simulink model "orbit"  (R2025b)
settings: Solver=ode45  StartTime=0.0  StopTime=endTime  FixedStep=1/60  MaxStep=10  RelTol=1e-10  AbsTol=1e-10
undefined symbols (not defined in the file or in its folder): panelY
libraries: aerolibutil x9, aerolibsatdyn x3, simulink_extras x2
settings Model: Creator=The MathWorks, Inc.  LastModifiedBy=axmal
settings OptimizationCC: ReuseModelBlockBuffer=off
settings ModelReferenceCC: EnableRefExpFcnMdlSchedulingChecks=on
settings RTWCC: GPUComputeCapability=3.5

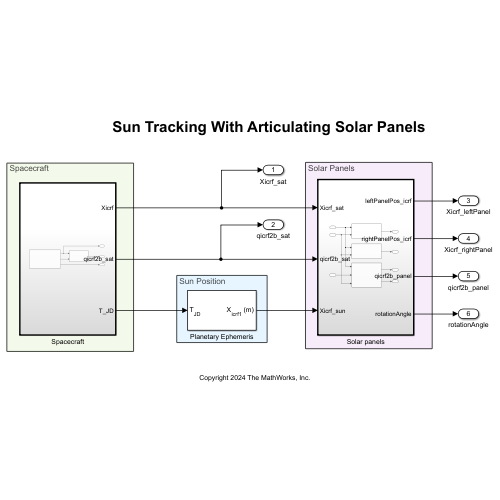
[thumbnail: Simulink's stored preview of the top-level diagram]
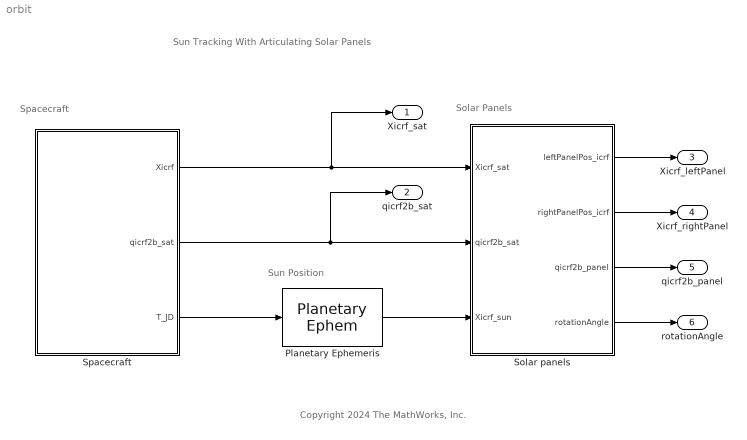
== system orbit ==
  note: Sun Position
  note: Spacecraft
  note: Sun Tracking With Articulating Solar Panels
  note: Copyright 2024 The MathWorks, Inc.
  note: Solar Panels
  Planetary Ephemeris : PlanetaryEphem  units=m,m/s  target=Sun  outputVelocity=off
  Solar panels : Subsystem  TreatAsAtomicUnit=on
  Spacecraft : Subsystem  TreatAsAtomicUnit=on
  Xicrf_sat : Outport
  qicrf2b_sat : Outport  Port=2
  Xicrf_leftPanel : Outport  Port=3
  Xicrf_rightPanel : Outport  Port=4
  qicrf2b_panel : Outport  Port=5
  rotationAngle : Outport  Port=6
  wires:
  Spacecraft/3(T_JD) -> Planetary Ephemeris/1
  Spacecraft/2(qicrf2b_sat) -> qicrf2b_sat/1, Solar panels/2(qicrf2b_sat)
  Solar panels/2(rightPanelPos_icrf) -> Xicrf_rightPanel/1
  Solar panels/3(qicrf2b_panel) -> qicrf2b_panel/1
  Spacecraft/1(Xicrf) -> Xicrf_sat/1, Solar panels/1(Xicrf_sat)
  Planetary Ephemeris/1 -> Solar panels/3(Xicrf_sun)
  Solar panels/1(leftPanelPos_icrf) -> Xicrf_leftPanel/1
  Solar panels/4(rotationAngle) -> rotationAngle/1

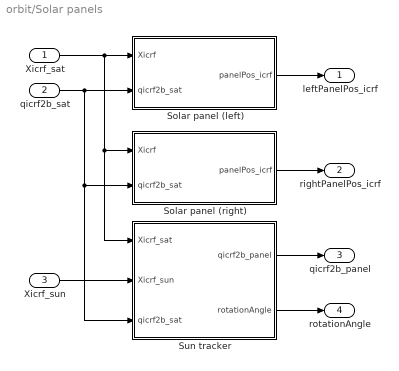
== system orbit/Solar panels ==
  Xicrf_sat : Inport
  qicrf2b_sat : Inport  Port=2
  Xicrf_sun : Inport  Port=3
  Solar panel (left) : Subsystem
  Solar panel (right) : Subsystem
  Sun tracker : Subsystem
  leftPanelPos_icrf : Outport
  rightPanelPos_icrf : Outport  Port=2
  qicrf2b_panel : Outport  Port=3
  rotationAngle : Outport  Port=4
  wires:
  Sun tracker/1(qicrf2b_panel) -> qicrf2b_panel/1
  Solar panel (right)/1(panelPos_icrf) -> rightPanelPos_icrf/1
  qicrf2b_sat/1 -> Sun tracker/3(qicrf2b_sat), Solar panel (right)/2(qicrf2b_sat), Solar panel (left)/2(qicrf2b_sat)
  Xicrf_sat/1 -> Sun tracker/1(Xicrf_sat), Solar panel (right)/1(Xicrf), Solar panel (left)/1(Xicrf)
  Solar panel (left)/1(panelPos_icrf) -> leftPanelPos_icrf/1
  Sun tracker/2(rotationAngle) -> rotationAngle/1
  Xicrf_sun/1 -> Sun tracker/2(Xicrf_sun)

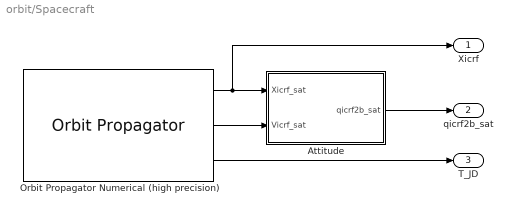
== system orbit/Spacecraft ==
  "Attitude " : Subsystem  TreatAsAtomicUnit=on
  Orbit Propagator Numerical (high precision) : OrbitPropagator  propagator=Numerical (high precision)  startDate=initialTimeJD  semiMajorAxis=semiMajorAxis  eccentricity=eccentricity  inclination=inclination  raan=rightAscensionOfAscendingNode  argPeriapsis=argumentOfPeriapsis  trueAnomaly=trueAnomaly  inertialPosition=[3649700.0 3308200.0 -4676600.0]  inertialVelocity=[-2750.8 6666.4 2573.4]  fixedPosition=[-4142689.0 -2676864.7 -4669861.6]  fixedVelocity=[1452.7 -6720.7 2568.1]  gravityModel=Point-mass  customR=3396200  customMu=4.305e13  customJ2=1.0826269e-03  customOmega=4.06125949e-3  useEOPs=off
  Xicrf : Outport
  qicrf2b_sat : Outport  Port=2
  T_JD : Outport  Port=3
  wires:
  Orbit Propagator Numerical (high precision)/3 -> T_JD/1
  Orbit Propagator Numerical (high precision)/1 -> Xicrf/1, "Attitude "/1(Xicrf_sat)
  Orbit Propagator Numerical (high precision)/2 -> "Attitude "/2(Vicrf_sat)
  "Attitude "/1(qicrf2b_sat) -> qicrf2b_sat/1

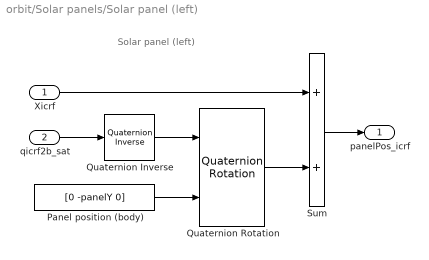
== system orbit/Solar panels/Solar panel (left) ==
  note: Solar panel (left)
  Xicrf : Inport
  qicrf2b_sat : Inport  Port=2
  Panel position (body) : Constant  Value=[0 -panelY 0]
  Quaternion Inverse : aerolibutil/Quaternion Inverse
  Quaternion Rotation : aerolibutil/Quaternion Rotation
  Sum : Sum
  panelPos_icrf : Outport
  wires:
  Quaternion Inverse/1 -> Quaternion Rotation/1
  Quaternion Rotation/1 -> Sum/2
  qicrf2b_sat/1 -> Quaternion Inverse/1
  Panel position (body)/1 -> Quaternion Rotation/2
  Xicrf/1 -> Sum/1
  Sum/1 -> panelPos_icrf/1

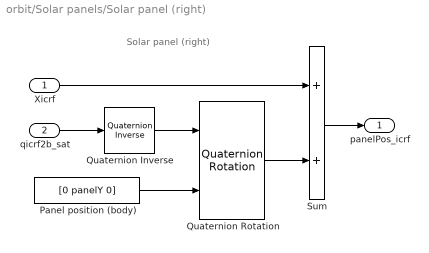
== system orbit/Solar panels/Solar panel (right) ==
  note: Solar panel (right)
  Xicrf : Inport
  qicrf2b_sat : Inport  Port=2
  Panel position (body) : Constant  Value=[0 panelY 0]
  Quaternion Inverse : aerolibutil/Quaternion Inverse
  Quaternion Rotation : aerolibutil/Quaternion Rotation
  Sum : Sum
  panelPos_icrf : Outport
  wires:
  Quaternion Inverse/1 -> Quaternion Rotation/1
  Quaternion Rotation/1 -> Sum/2
  qicrf2b_sat/1 -> Quaternion Inverse/1
  Panel position (body)/1 -> Quaternion Rotation/2
  Xicrf/1 -> Sum/1
  Sum/1 -> panelPos_icrf/1

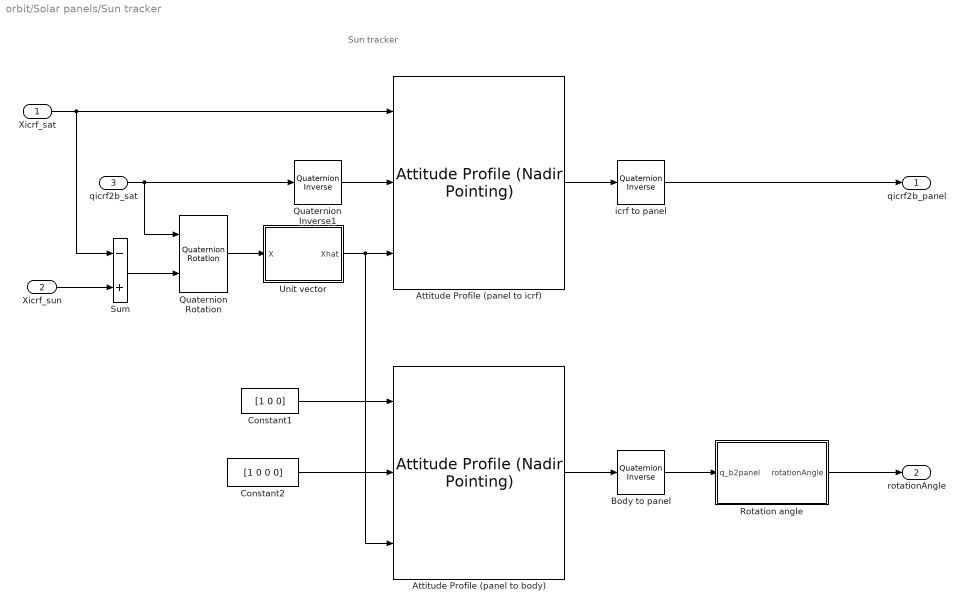
== system orbit/Solar panels/Sun tracker ==
  note: Sun tracker
  Xicrf_sat : Inport
  Xicrf_sun : Inport  Port=2
  qicrf2b_sat : Inport  Port=3
  Attitude Profile (panel to body) : aerolibsatdyn/Attitude Profile (Nadir Pointing)  outputError=off  outputFinalAttitude=on  portFrame=ICRF  pointingMode=Custom  celestialTarget=Sun  tunablePointing=off  primaryAlignmentSrc=Dialog  primaryAlignment=[0 1 0]  secondaryAlignmentSrc=Dialog  secondaryAlignment=[0 0 1]  constraintFrame=Body-frame  primaryConstraintSrc=Dialog  primaryConstraint=[0 1 0]  secondaryConstraintSrc=Port  secondaryConstraint=[0 1 0]
  Attitude Profile (panel to icrf) : aerolibsatdyn/Attitude Profile (Nadir Pointing)  outputError=off  outputFinalAttitude=on  portFrame=ICRF  pointingMode=Custom  celestialTarget=Sun  tunablePointing=off  primaryAlignmentSrc=Dialog  primaryAlignment=[0 1 0]  secondaryAlignmentSrc=Dialog  secondaryAlignment=[0 0 1]  constraintFrame=Body-frame  primaryConstraintSrc=Dialog  primaryConstraint=[0 1 0]  secondaryConstraintSrc=Port  secondaryConstraint=[0 1 0]
  Body to panel : aerolibutil/Quaternion Inverse
  Constant1 : Constant  Value=[1 0 0]
  Constant2 : Constant  Value=[1 0 0 0]
  Quaternion Inverse1 : aerolibutil/Quaternion Inverse
  Quaternion Rotation : aerolibutil/Quaternion Rotation
  Rotation angle : Subsystem
  Sum : Sum  Inputs=-+
  Unit vector : Subsystem
  icrf to panel : aerolibutil/Quaternion Inverse
  qicrf2b_panel : Outport
  rotationAngle : Outport  Port=2
  wires:
  icrf to panel/1 -> qicrf2b_panel/1
  qicrf2b_sat/1 -> Quaternion Rotation/1, Quaternion Inverse1/1
  Quaternion Inverse1/1 -> Attitude Profile (panel to icrf)/2
  Xicrf_sat/1 -> Sum/1, Attitude Profile (panel to icrf)/1
  Attitude Profile (panel to icrf)/1 -> icrf to panel/1
  Quaternion Rotation/1 -> Unit vector/1(X)
  Attitude Profile (panel to body)/1 -> Body to panel/1
  Constant1/1 -> Attitude Profile (panel to body)/1
  Unit vector/1(Xhat) -> Attitude Profile (panel to body)/3, Attitude Profile (panel to icrf)/3
  Constant2/1 -> Attitude Profile (panel to body)/2
  Body to panel/1 -> Rotation angle/1(q_b2panel)
  Rotation angle/1(rotationAngle) -> rotationAngle/1
  Xicrf_sun/1 -> Sum/2
  Sum/1 -> Quaternion Rotation/2

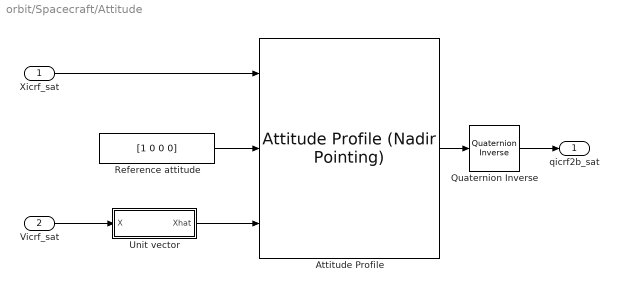
== system orbit/Spacecraft/Attitude  ==
  Xicrf_sat : Inport
  Vicrf_sat : Inport  Port=2
  Attitude Profile : aerolibsatdyn/Attitude Profile (Nadir Pointing)  outputError=off  outputFinalAttitude=on  portFrame=ICRF  pointingMode=Point at nadir  celestialTarget=Sun  tunablePointing=off  primaryAlignmentSrc=Dialog  primaryAlignment=[0 0 1]  secondaryAlignmentSrc=Dialog  secondaryAlignment=[1 0 0]  constraintFrame=ICRF  primaryConstraintSrc=Port  primaryConstraint=[1 0 0]  secondaryConstraintSrc=Port  secondaryConstraint=[0 0 1]
  Quaternion Inverse : aerolibutil/Quaternion Inverse
  Reference attitude : Constant  Value=[1 0 0 0]
  Unit vector : Subsystem
  qicrf2b_sat : Outport
  wires:
  Quaternion Inverse/1 -> qicrf2b_sat/1
  Vicrf_sat/1 -> Unit vector/1(X)
  Attitude Profile/1 -> Quaternion Inverse/1
  Reference attitude/1 -> Attitude Profile/2
  Unit vector/1(Xhat) -> Attitude Profile/3
  Xicrf_sat/1 -> Attitude Profile/1

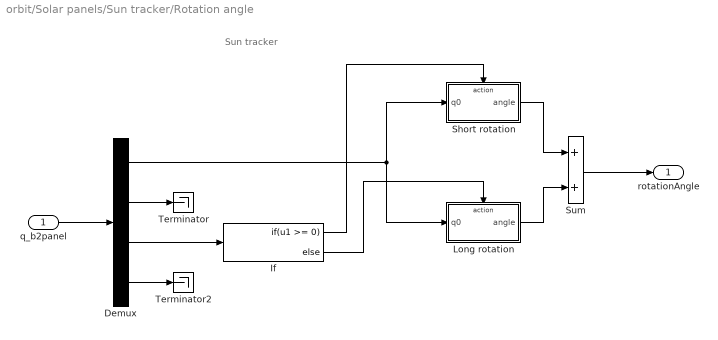
== system orbit/Solar panels/Sun tracker/Rotation angle ==
  note: Sun tracker
  q_b2panel : Inport
  Demux : Demux
  If : If  IfExpression=u1 >= 0
  Long rotation : Subsystem  TreatAsAtomicUnit=on
  Short rotation : Subsystem  TreatAsAtomicUnit=on
  Sum : Sum
  Terminator : Terminator
  Terminator2 : Terminator
  rotationAngle : Outport
  wires:
  Long rotation/1(angle) -> Sum/2
  Short rotation/1(angle) -> Sum/1
  Demux/1 -> Short rotation/1(q0), Long rotation/1(q0)
  Demux/3 -> If/1
  If/2 -> Long rotation/Action
  If/1 -> Short rotation/Action
  Sum/1 -> rotationAngle/1
  q_b2panel/1 -> Demux/1
  Demux/2 -> Terminator/1
  Demux/4 -> Terminator2/1

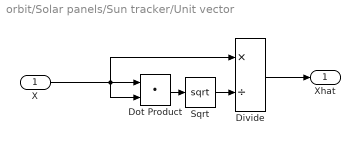
== system orbit/Solar panels/Sun tracker/Unit vector ==
  X : Inport
  Divide : Product  Inputs=*/
  Dot Product : DotProduct  OutDataTypeStr=Inherit: Inherit via internal rule
  Sqrt : Sqrt
  Xhat : Outport
  wires:
  Dot Product/1 -> Sqrt/1
  X/1 -> Divide/1, Dot Product/2, Dot Product/1
  Divide/1 -> Xhat/1
  Sqrt/1 -> Divide/2

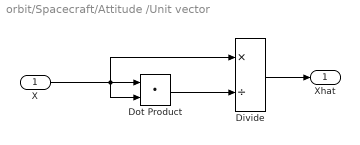
== system orbit/Spacecraft/Attitude /Unit vector ==
  X : Inport
  Divide : Product  Inputs=*/
  Dot Product : DotProduct  OutDataTypeStr=Inherit: Inherit via internal rule
  Xhat : Outport
  wires:
  Dot Product/1 -> Divide/2
  X/1 -> Divide/1, Dot Product/2, Dot Product/1
  Divide/1 -> Xhat/1

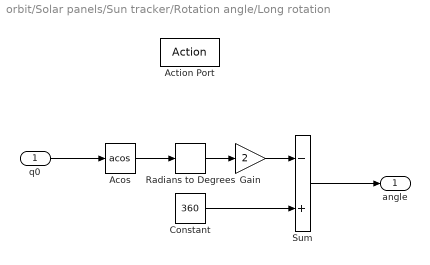
== system orbit/Solar panels/Sun tracker/Rotation angle/Long rotation ==
  q0 : Inport
  Action Port : ActionPort  ActionPortLabel=else
  Acos : Trigonometry  Operator=acos
  Constant : Constant  Value=360
  Gain : Gain  Gain=2
  Radians to Degrees : simulink_extras/Transformations/Radians to Degrees
  Sum : Sum  Inputs=-+
  angle : Outport  OutputWhenDisabled=reset  InitialOutput=0
  wires:
  Acos/1 -> Radians to Degrees/1
  q0/1 -> Acos/1
  Radians to Degrees/1 -> Gain/1
  Constant/1 -> Sum/2
  Sum/1 -> angle/1
  Gain/1 -> Sum/1

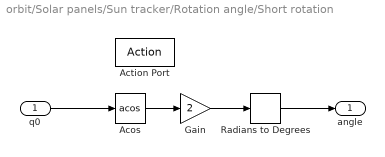
== system orbit/Solar panels/Sun tracker/Rotation angle/Short rotation ==
  q0 : Inport
  Action Port : ActionPort  ActionPortLabel=if(u1 >= 0)
  Acos : Trigonometry  Operator=acos
  Gain : Gain  Gain=2
  Radians to Degrees : simulink_extras/Transformations/Radians to Degrees
  angle : Outport  OutputWhenDisabled=reset  InitialOutput=0
  wires:
  q0/1 -> Acos/1
  Acos/1 -> Gain/1
  Radians to Degrees/1 -> angle/1
  Gain/1 -> Radians to Degrees/1
